simulink model "Attitude_Estimator"  (Simulink 9.0)
settings: Solver=FixedStepDiscrete  StartTime=0.0  StopTime=tsim  FixedStep=te  RelTol=1e-3
values from neighbouring files (symbols this model uses):
  FILTER_KI = 0.1    [Attitude_Estimator_parameters.m]
  FILTER_KP = 1    [Attitude_Estimator_parameters.m]
  Gravity_Err_Threshold = 0.01    [Attitude_Estimator_parameters.m]
  Immobility_Threshold = 0.2    [Attitude_Estimator_parameters.m]
  Immobility_Time_Confirmation = 0.5    [Attitude_Estimator_parameters.m]
  Q_EST_INIT = [0 0 0 1]    [Attitude_Estimator_parameters.m]
  te = 0.01    [Attitude_Estimator_parameters.m]
undefined symbols (not defined in the file or in its folder): DiscIntNeverNeededParam
libraries: simulink x5
settings Model: Creator=sam  LastModifiedBy=William  ExtModeTrigDuration=2
settings DataIOCC: SaveFormat=Dataset
settings OptimizationCC: DefaultParameterBehavior=Inlined  DefaultUnderspecifiedDataType=single  PassReuseOutputArgsThreshold=0  LifeSpan=auto  MaxStackSize=64
settings DebuggingCC: UnderspecifiedInitializationDetection=Simplified  MergeDetectMultiDrivingBlocksExec=error  ParameterPrecisionLossMsg=none  ParameterTunabilityLossMsg=error
settings HardwareCC: ProdBitPerPointer=64  ProdBitPerSizeT=64  ProdBitPerPtrDiffT=64  ProdLargestAtomicFloat=Float  ProdIntDivRoundTo=Zero  ProdEndianess=LittleEndian  ProdWordSize=64  ProdHWDeviceType=Intel->x86-64 (Windows64)
settings ModelReferenceCC: PropagateSignalLabelsOutOfModel=on
settings SFSimCC: MATLABDynamicMemAlloc=off
settings RTWCC: GenerateReport=on  Toolchain=Arduino ARM  BuildConfiguration=Faster Runs  LaunchReport=on  RTWCompilerOptimization=on
settings CodeAppCC: ForceParamTrailComments=on  MaxIdLength=95  OperatorAnnotations=on  MATLABSourceComments=on
settings ConfigComp: CovScope=ReferencedModels  CovIncludeTopModel=off  CovSaveName=covdata_decision  CovMetricSettings=dcmw  CovHTMLOptions=-sRT=1 -sVT=0 -aTS=1 -bRG=1 -bTC=1 -hTR=0 -nFC=0 -nFD=1 -scm=1 -bcm=1 -xEv=0 -xEM=0  CovNameIncrementing=on  CovOutputDir=../reports/slcov_output/$ModelName$

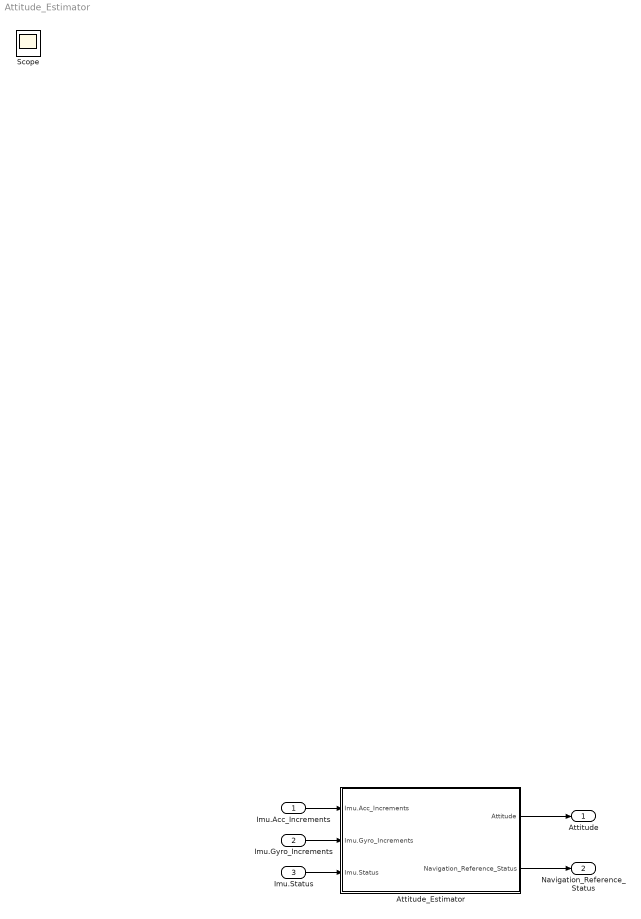
== system Attitude_Estimator ==
  Imu.Acc_Increments : Inport  OutDataTypeStr=single  PortDimensions=3
  Imu.Gyro_Increments : Inport  Port=2  PortDimensions=3
  Imu.Status : Inport  Port=3  PortDimensions=1
  Attitude_Estimator : Subsystem
  Attitude : Outport  PortDimensions=5
  Navigation_Reference_Status : Outport  Port=2  PortDimensions=1
  Scope : Scope
  wires:
  Attitude_Estimator/1(Attitude) -> Attitude/1
  Imu.Acc_Increments/1 -> Attitude_Estimator/1(Imu.Acc_Increments)
  Attitude_Estimator/2(Navigation_Reference_Status) -> Navigation_Reference_Status/1
  Imu.Gyro_Increments/1 -> Attitude_Estimator/2(Imu.Gyro_Increments)
  Imu.Status/1 -> Attitude_Estimator/3(Imu.Status)

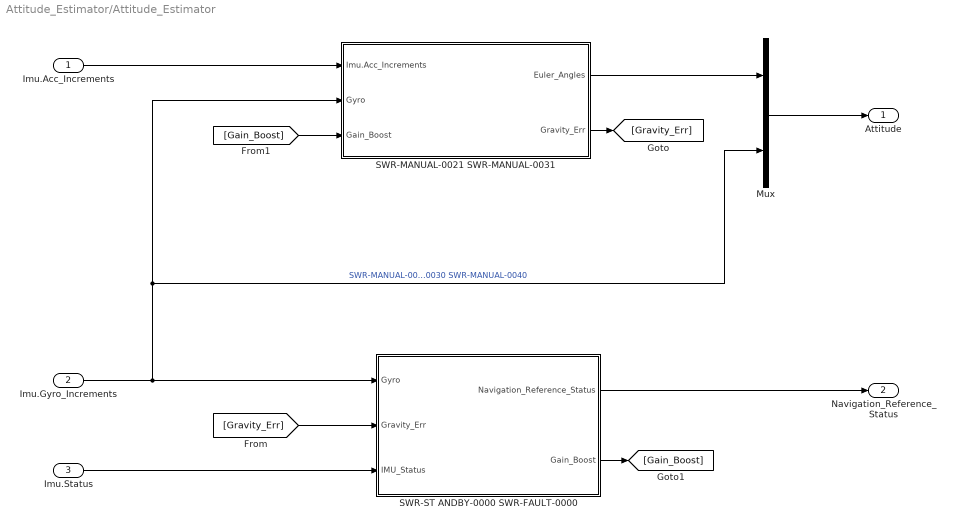
== system Attitude_Estimator/Attitude_Estimator ==
  Imu.Acc_Increments : Inport  OutDataTypeStr=single  PortDimensions=3
  Imu.Gyro_Increments : Inport  Port=2  OutDataTypeStr=single  PortDimensions=3
  Imu.Status : Inport  Port=3  OutDataTypeStr=uint8  PortDimensions=1
  Mux : Mux  Inputs=2
  SWR-MANUAL-0021 SWR-MANUAL-0031 : Subsystem
  SWR-ST	ANDBY-0000 SWR-FAULT-0000 : Subsystem
  Attitude : Outport  OutDataTypeStr=single  PortDimensions=5
  Navigation_Reference_Status : Outport  Port=2  OutDataTypeStr=uint8  PortDimensions=1
  wires:
  Imu.Gyro_Increments/1 -> SWR-ST	ANDBY-0000 SWR-FAULT-0000/1(Gyro), SWR-MANUAL-0021 SWR-MANUAL-0031/2(Gyro), Mux/2  "SWR-MANUAL-0020 SWR-MANUAL-0030 SWR-MANUAL-0040"
  [Gravity_Err] -> SWR-ST	ANDBY-0000 SWR-FAULT-0000/2(Gravity_Err)
  Imu.Status/1 -> SWR-ST	ANDBY-0000 SWR-FAULT-0000/3(IMU_Status)
  SWR-ST	ANDBY-0000 SWR-FAULT-0000/1(Navigation_Reference_Status) -> Navigation_Reference_Status/1
  SWR-ST	ANDBY-0000 SWR-FAULT-0000/2(Gain_Boost) -> [Gain_Boost]
  Mux/1 -> Attitude/1
  Imu.Acc_Increments/1 -> SWR-MANUAL-0021 SWR-MANUAL-0031/1(Imu.Acc_Increments)
  SWR-MANUAL-0021 SWR-MANUAL-0031/2(Gravity_Err) -> [Gravity_Err]
  SWR-MANUAL-0021 SWR-MANUAL-0031/1(Euler_Angles) -> Mux/1
  [Gain_Boost] -> SWR-MANUAL-0021 SWR-MANUAL-0031/3(Gain_Boost)

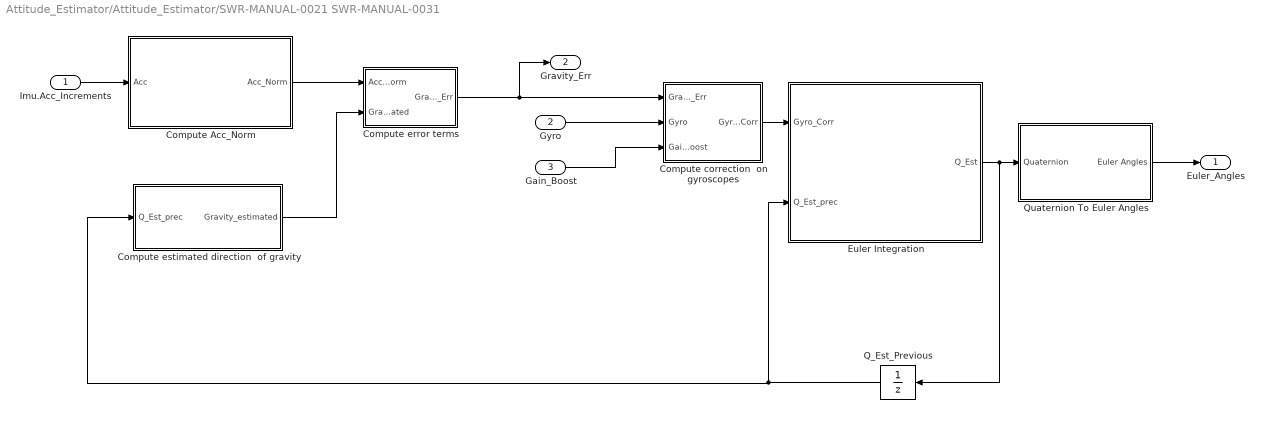
== system Attitude_Estimator/Attitude_Estimator/SWR-MANUAL-0021 SWR-MANUAL-0031 ==
  Imu.Acc_Increments : Inport  OutDataTypeStr=single  PortDimensions=3
  Gyro : Inport  Port=2
  Gain_Boost : Inport  Port=3
  Compute Acc_Norm : Subsystem
  Compute correction  on gyroscopes : Subsystem
  Compute error terms : Subsystem
  Compute estimated direction  of gravity : Subsystem
  Euler Integration : Subsystem
  Q_Est_Previous : UnitDelay  InitialCondition=Q_EST_INIT  SampleTime=te
  Quaternion To Euler Angles : Subsystem
  Euler_Angles : Outport
  Gravity_Err : Outport  Port=2  OutDataTypeStr=single  PortDimensions=3
  wires:
  Euler Integration/1(Q_Est) -> Quaternion To Euler Angles/1(Quaternion), Q_Est_Previous/1
  Compute estimated direction  of gravity/1(Gravity_estimated) -> Compute error terms/2(Gravity_estimated)
  Compute correction  on gyroscopes/1(Gyro_Corr) -> Euler Integration/1(Gyro_Corr)
  Compute Acc_Norm/1(Acc_Norm) -> Compute error terms/1(Acc_Norm)
  Compute error terms/1(Gravity_Err) -> Gravity_Err/1, Compute correction  on gyroscopes/1(Gravity_Err)
  Imu.Acc_Increments/1 -> Compute Acc_Norm/1(Acc)
  Q_Est_Previous/1 -> Compute estimated direction  of gravity/1(Q_Est_prec), Euler Integration/2(Q_Est_prec)
  Quaternion To Euler Angles/1(Euler Angles) -> Euler_Angles/1
  Gain_Boost/1 -> Compute correction  on gyroscopes/3(Gain_Boost)
  Gyro/1 -> Compute correction  on gyroscopes/2(Gyro)

== system Attitude_Estimator/Attitude_Estimator/SWR-ST	ANDBY-0000 SWR-FAULT-0000 ==
  Gyro : Inport
  Gravity_Err : Inport  Port=2
  IMU_Status : Inport  Port=3
  SWR-ST	ANDBY-0000 SWR-FAULT-0000 : Subsystem
  SWR-STANDBY-0000 : Subsystem
  Navigation_Reference_Status : Outport
  Gain_Boost : Outport  Port=2  PortDimensions=1
  wires:
  Gyro/1 -> SWR-STANDBY-0000/2(Gyro)
  Gravity_Err/1 -> SWR-STANDBY-0000/3(Gravity_Err)
  SWR-STANDBY-0000/2(Gain_Boost) -> Gain_Boost/1
  IMU_Status/1 -> SWR-STANDBY-0000/1(IMU_Status), SWR-ST	ANDBY-0000 SWR-FAULT-0000/1(Imu_Status)
  SWR-STANDBY-0000/1(Alignment_OK) -> SWR-ST	ANDBY-0000 SWR-FAULT-0000/2(Alignment_OK)
  SWR-ST	ANDBY-0000 SWR-FAULT-0000/1(Navigation_Reference_Status) -> Navigation_Reference_Status/1

== system Attitude_Estimator/Attitude_Estimator/SWR-MANUAL-0021 SWR-MANUAL-0031/Compute Acc_Norm ==
  Acc : Inport  PortDimensions=3
  Normalize 3D Vector : Subsystem
  Acc_Norm : Outport  OutDataTypeStr=single  PortDimensions=3
  wires:
  Acc/1 -> Normalize 3D Vector/1(Acc)
  Normalize 3D Vector/1(Acc_Norm) -> Acc_Norm/1

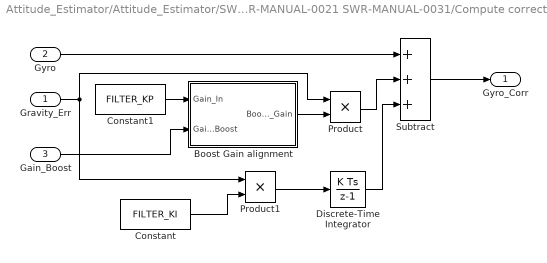
== system Attitude_Estimator/Attitude_Estimator/SWR-MANUAL-0021 SWR-MANUAL-0031/Compute correction  on gyroscopes ==
  Gravity_Err : Inport  PortDimensions=3
  Gyro : Inport  Port=2  PortDimensions=3
  Gain_Boost : Inport  Port=3  PortDimensions=1
  Boost Gain alignment : Subsystem
  Constant : Constant  Value=FILTER_KI  OutDataTypeStr=single
  Constant1 : Constant  Value=FILTER_KP  OutDataTypeStr=single
  Discrete-Time Integrator : DiscreteIntegrator  InitialConditionSetting=State (most efficient)  SampleTime=te  ICPrevOutput=DiscIntNeverNeededParam  ICPrevScaledInput=DiscIntNeverNeededParam
  Product : Product
  Product1 : Product
  Subtract : Sum  Inputs=+++
  Gyro_Corr : Outport  PortDimensions=3
  wires:
  Gyro/1 -> Subtract/1
  Subtract/1 -> Gyro_Corr/1
  Gravity_Err/1 -> Product1/1, Product/1
  Product/1 -> Subtract/2
  Constant/1 -> Product1/2
  Product1/1 -> Discrete-Time Integrator/1
  Discrete-Time Integrator/1 -> Subtract/3
  Boost Gain alignment/1(Boosted_Gain) -> Product/2
  Constant1/1 -> Boost Gain alignment/1(Gain_In)
  Gain_Boost/1 -> Boost Gain alignment/2(Gain_Boost)

== system Attitude_Estimator/Attitude_Estimator/SWR-MANUAL-0021 SWR-MANUAL-0031/Compute error terms ==
  Acc_Norm : Inport  PortDimensions=3
  Gravity_estimated : Inport  Port=2  PortDimensions=3
  Cross Product : Subsystem
  Gravity_Err : Outport  PortDimensions=3
  wires:
  Gravity_estimated/1 -> Cross Product/1(Vec1)
  Acc_Norm/1 -> Cross Product/2(Vec2)
  Cross Product/1(Prod_Vec) -> Gravity_Err/1

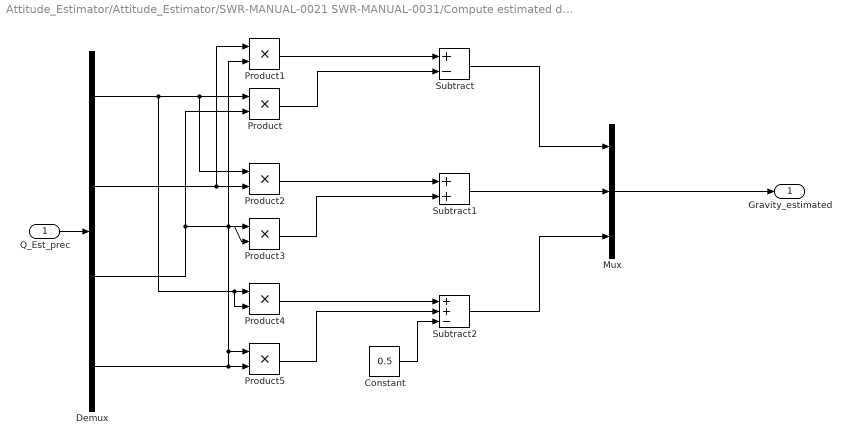
== system Attitude_Estimator/Attitude_Estimator/SWR-MANUAL-0021 SWR-MANUAL-0031/Compute estimated direction  of gravity ==
  Q_Est_prec : Inport  PortDimensions=4
  Constant : Constant  Value=0.5  OutDataTypeStr=single
  Demux : Demux
  Mux : Mux  Inputs=3
  Product{,1..5} (6 alike) : Product
  Subtract : Sum  Inputs=+-
  Subtract1 : Sum
  Subtract2 : Sum  Inputs=++-
  Gravity_estimated : Outport
  wires:
  Q_Est_prec/1 -> Demux/1
  Demux/2 -> Product2/2, Product1/1
  Demux/4 -> Product5/1, Product3/2, Product1/2, Product5/2
  Demux/1 -> Product/1, Product2/1, Product4/2, Product4/1
  Demux/3 -> Product/2, Product3/1
  Product1/1 -> Subtract/1
  Product/1 -> Subtract/2
  Product2/1 -> Subtract1/1
  Product3/1 -> Subtract1/2
  Product4/1 -> Subtract2/1
  Product5/1 -> Subtract2/2
  Constant/1 -> Subtract2/3
  Subtract/1 -> Mux/1
  Subtract1/1 -> Mux/2
  Subtract2/1 -> Mux/3
  Mux/1 -> Gravity_estimated/1

== system Attitude_Estimator/Attitude_Estimator/SWR-MANUAL-0021 SWR-MANUAL-0031/Euler Integration ==
  Gyro_Corr : Inport  PortDimensions=3
  Q_Est_prec : Inport  Port=2  PortDimensions=4
  Add : Sum
  Compute Kinematic Propagation Quaternion : Subsystem
  Compute Unit Quaternion : Subsystem
  Gain : Gain  Gain=0.5*te  OutDataTypeStr=single
  Q_Est : Outport  PortDimensions=4
  wires:
  Compute Unit Quaternion/1(Qn) -> Q_Est/1
  Q_Est_prec/1 -> Add/1, Compute Kinematic Propagation Quaternion/1(Q_Est_Prec)
  Gyro_Corr/1 -> Compute Kinematic Propagation Quaternion/2(W_F inal)
  Compute Kinematic Propagation Quaternion/1(Kin_Prop_Quat) -> Gain/1
  Gain/1 -> Add/2
  Add/1 -> Compute Unit Quaternion/1(Q)

== system Attitude_Estimator/Attitude_Estimator/SWR-MANUAL-0021 SWR-MANUAL-0031/Quaternion To Euler Angles ==
  Quaternion : Inport  PortDimensions=4
  Compute Pitch : Subsystem
  "Compute Roll " : Subsystem
  Mux : Mux  Inputs=2
  Euler Angles : Outport  PortDimensions=2
  wires:
  Mux/1 -> Euler Angles/1
  "Compute Roll "/1(Roll) -> Mux/1
  Quaternion/1 -> Compute Pitch/1(Quaternion), "Compute Roll "/1(Quaternion)
  Compute Pitch/1(Pitch) -> Mux/2

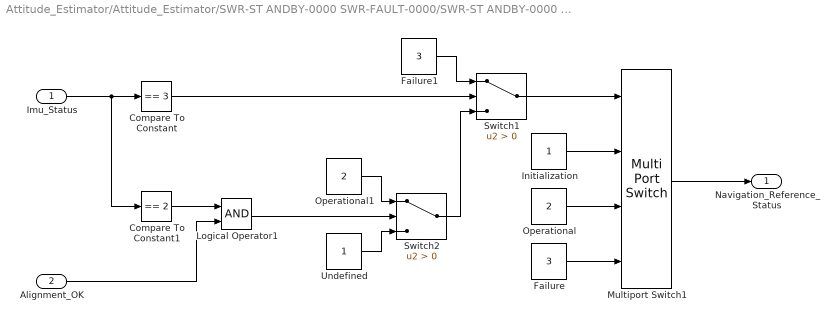
== system Attitude_Estimator/Attitude_Estimator/SWR-ST	ANDBY-0000 SWR-FAULT-0000/SWR-ST	ANDBY-0000 SWR-FAULT-0000 ==
  Imu_Status : Inport
  Alignment_OK : Inport  Port=2
  Compare To Constant : simulink/Logic and Bit Operations/Compare To Constant  relop===  const=3  OutDataTypeStr=boolean
  Compare To Constant1 : simulink/Logic and Bit Operations/Compare To Constant  relop===  const=2  OutDataTypeStr=boolean
  Failure : Constant  Value=3  OutDataTypeStr=uint8
  Failure1 : Constant  Value=3  OutDataTypeStr=uint8
  Initialization : Constant  OutDataTypeStr=uint8
  Logical Operator1 : Logic  AllPortsSameDT=off  OutDataTypeStr=boolean
  Multiport Switch1 : MultiPortSwitch  DiagnosticForDefault=None
  Operational : Constant  Value=2  OutDataTypeStr=uint8
  Operational1 : Constant  Value=2  OutDataTypeStr=uint8
  Switch1 : Switch  Criteria=u2 > Threshold
  Switch2 : Switch  Criteria=u2 > Threshold
  Undefined : Constant  OutDataTypeStr=uint8
  Navigation_Reference_Status : Outport
  wires:
  Logical Operator1/1 -> Switch2/2
  Compare To Constant1/1 -> Logical Operator1/1
  Undefined/1 -> Switch2/3
  Switch1/1 -> Multiport Switch1/1
  Failure1/1 -> Switch1/1
  Operational1/1 -> Switch2/1
  Switch2/1 -> Switch1/3
  Multiport Switch1/1 -> Navigation_Reference_Status/1
  Initialization/1 -> Multiport Switch1/2
  Operational/1 -> Multiport Switch1/3
  Failure/1 -> Multiport Switch1/4
  Alignment_OK/1 -> Logical Operator1/2
  Compare To Constant/1 -> Switch1/2
  Imu_Status/1 -> Compare To Constant/1, Compare To Constant1/1

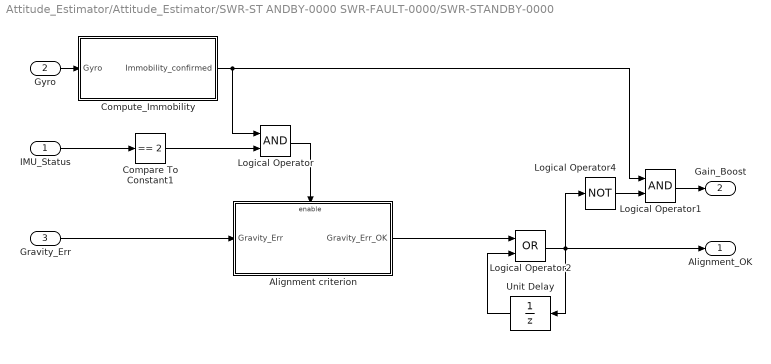
== system Attitude_Estimator/Attitude_Estimator/SWR-ST	ANDBY-0000 SWR-FAULT-0000/SWR-STANDBY-0000 ==
  IMU_Status : Inport
  Gyro : Inport  Port=2
  Gravity_Err : Inport  Port=3
  Alignment criterion : Subsystem  TreatAsAtomicUnit=on
  Compare To Constant1 : simulink/Logic and Bit Operations/Compare To Constant  relop===  const=2  OutDataTypeStr=boolean
  Compute_Immobility : Subsystem
  Logical Operator : Logic  AllPortsSameDT=off  OutDataTypeStr=boolean
  Logical Operator1 : Logic  AllPortsSameDT=off  OutDataTypeStr=boolean
  Logical Operator2 : Logic  Operator=OR  AllPortsSameDT=off  OutDataTypeStr=boolean
  Logical Operator4 : Logic  Operator=NOT  AllPortsSameDT=off  OutDataTypeStr=boolean
  Unit Delay : UnitDelay  SampleTime=te
  Alignment_OK : Outport  PortDimensions=1
  Gain_Boost : Outport  Port=2  PortDimensions=1
  wires:
  Gyro/1 -> Compute_Immobility/1(Gyro)
  Compute_Immobility/1(Immobility_confirmed) -> Logical Operator1/1, Logical Operator/1
  Logical Operator2/1 -> Alignment_OK/1, Unit Delay/1, Logical Operator4/1
  Unit Delay/1 -> Logical Operator2/2
  Gravity_Err/1 -> Alignment criterion/1(Gravity_Err)
  Logical Operator1/1 -> Gain_Boost/1
  Logical Operator4/1 -> Logical Operator1/2
  Logical Operator/1 -> Alignment criterion/Enable
  IMU_Status/1 -> Compare To Constant1/1
  Compare To Constant1/1 -> Logical Operator/2
  Alignment criterion/1(Gravity_Err_OK) -> Logical Operator2/1

== system Attitude_Estimator/Attitude_Estimator/SWR-MANUAL-0021 SWR-MANUAL-0031/Compute Acc_Norm/Normalize 3D Vector ==
  Acc : Inport  PortDimensions=3
  Compare To Constant : simulink/Logic and Bit Operations/Compare To Constant  relop===  const=0.0  OutDataTypeStr=boolean
  Constant : Constant  OutDataTypeStr=single
  Divide : Product  Inputs=*/
  Switch : Switch  Criteria=u2 > Threshold
  Vect 3D Norm : Subsystem
  Acc_Norm : Outport  PortDimensions=3
  wires:
  Acc/1 -> Vect 3D Norm/1(Vect_3D), Divide/1
  Vect 3D Norm/1(Vect_3D_Norm) -> Compare To Constant/1, Switch/3
  Compare To Constant/1 -> Switch/2
  Switch/1 -> Divide/2
  Divide/1 -> Acc_Norm/1
  Constant/1 -> Switch/1

== system Attitude_Estimator/Attitude_Estimator/SWR-MANUAL-0021 SWR-MANUAL-0031/Compute correction  on gyroscopes/Boost Gain alignment ==
  Gain_In : Inport  PortDimensions=1
  Gain_Boost : Inport  Port=2  PortDimensions=1
  Gain : Gain  Gain=10
  Switch : Switch  Criteria=u2 > Threshold
  Boosted_Gain : Outport  PortDimensions=1
  wires:
  Switch/1 -> Boosted_Gain/1
  Gain_In/1 -> Gain/1, Switch/3
  Gain_Boost/1 -> Switch/2
  Gain/1 -> Switch/1

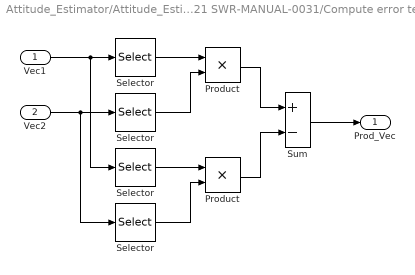
== system Attitude_Estimator/Attitude_Estimator/SWR-MANUAL-0021 SWR-MANUAL-0031/Compute error terms/Cross Product ==
  Vec1 : Inport  PortDimensions=3
  Vec2 : Inport  Port=2  PortDimensions=3
  " Selector " : Selector  IndexMode=Zero-based  InputPortWidth=3  IndexOptions=Index vector (dialog)  Indices=[1 2 0]  OutputSizes=1
  Product : Product  RndMeth=Zero  InputSameDT=on  OutDataTypeStr=Inherit: Same as first input
  "Product " : Product  RndMeth=Zero  InputSameDT=on  OutDataTypeStr=Inherit: Same as first input
  Selector : Selector  IndexMode=Zero-based  InputPortWidth=3  IndexOptions=Index vector (dialog)  Indices=[1 2 0]  OutputSizes=1
  "Selector " : Selector  IndexMode=Zero-based  InputPortWidth=3  IndexOptions=Index vector (dialog)  Indices=[2 0 1]  OutputSizes=1
  "Selector  " : Selector  IndexMode=Zero-based  InputPortWidth=3  IndexOptions=Index vector (dialog)  Indices=[2 0 1]  OutputSizes=1
  Sum : Sum  Inputs=+-  InputSameDT=on  OutDataTypeStr=Inherit: Same as first input
  Prod_Vec : Outport  PortDimensions=3
  wires:
  "Selector  "/1 -> "Product "/1
  Selector/1 -> Product/1
  Sum/1 -> Prod_Vec/1
  " Selector "/1 -> "Product "/2
  "Product "/1 -> Sum/2
  "Selector "/1 -> Product/2
  Product/1 -> Sum/1
  Vec1/1 -> "Selector  "/1, Selector/1
  Vec2/1 -> " Selector "/1, "Selector "/1

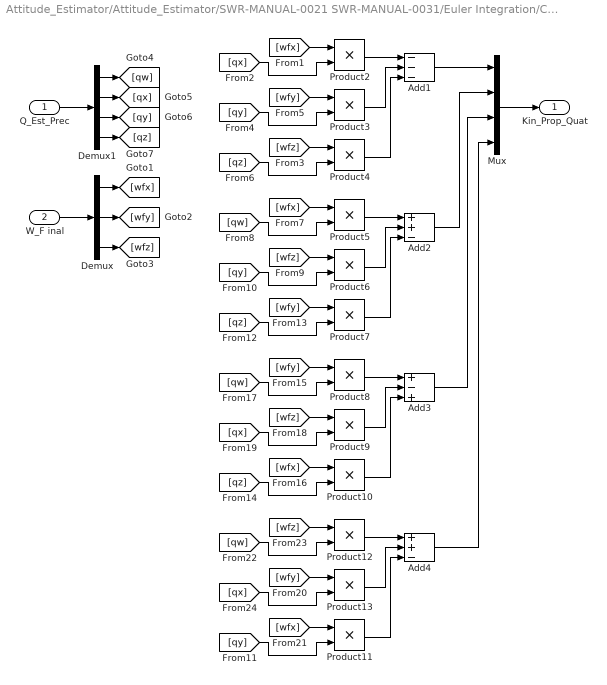
== system Attitude_Estimator/Attitude_Estimator/SWR-MANUAL-0021 SWR-MANUAL-0031/Euler Integration/Compute Kinematic Propagation Quaternion ==
  Q_Est_Prec : Inport  PortDimensions=4
  W_F inal : Inport  Port=2  PortDimensions=3
  Add1 : Sum  Inputs=---
  Add2 : Sum  Inputs=++-
  Add3 : Sum  Inputs=+-+
  Add4 : Sum  Inputs=++-
  Demux : Demux  Outputs=3
  Demux1 : Demux
  Mux : Mux
  Product{2..13} (12 alike) : Product
  Kin_Prop_Quat : Outport  PortDimensions=4
  wires:
  [wfx] -> Product11/1
  [wfz] -> Product12/1
  Demux1/3 -> [qy]
  Add2/1 -> Mux/2
  [wfx] -> Product10/1
  Product10/1 -> Add3/3
  [wfz] -> Product6/1
  Demux1/2 -> [qx]
  [wfy] -> Product7/1
  Demux/3 -> [wfz]
  Product11/1 -> Add4/3
  [qw] -> Product8/2
  Demux/1 -> [wfx]
  Add4/1 -> Mux/4
  Product5/1 -> Add2/1
  Q_Est_Prec/1 -> Demux1/1
  [wfx] -> Product2/1
  Add3/1 -> Mux/3
  Product7/1 -> Add2/3
  [wfz] -> Product9/1
  Product4/1 -> Add1/3
  [qz] -> Product7/2
  Product9/1 -> Add3/2
  Product3/1 -> Add1/2
  Product2/1 -> Add1/1
  Product6/1 -> Add2/2
  [qw] -> Product12/2
  Demux1/1 -> [qw]
  [qy] -> Product11/2
  [qy] -> Product6/2
  Product12/1 -> Add4/1
  [qx] -> Product9/2
  [qz] -> Product10/2
  Demux1/4 -> [qz]
  [wfy] -> Product13/1
  Product8/1 -> Add3/1
  [qw] -> Product5/2
  [qy] -> Product3/2
  [wfx] -> Product5/1
  Product13/1 -> Add4/2
  Add1/1 -> Mux/1
  Mux/1 -> Kin_Prop_Quat/1
  [qx] -> Product13/2
  Demux/2 -> [wfy]
  W_F inal/1 -> Demux/1
  [qx] -> Product2/2
  [wfy] -> Product8/1
  [wfy] -> Product3/1
  [wfz] -> Product4/1
  [qz] -> Product4/2

== system Attitude_Estimator/Attitude_Estimator/SWR-MANUAL-0021 SWR-MANUAL-0031/Euler Integration/Compute Unit Quaternion ==
  Q : Inport  PortDimensions=4
  Compare To Constant : simulink/Logic and Bit Operations/Compare To Constant  relop===  const=0  OutDataTypeStr=uint8
  Constant : Constant  OutDataTypeStr=single
  Divide : Product  Inputs=*/  OutDataTypeStr=Inherit: Same as first input
  Quaternion Norm : Subsystem
  Switch : Switch  Criteria=u2 > Threshold
  Qn : Outport  PortDimensions=4
  wires:
  Q/1 -> Divide/1, Quaternion Norm/1(Q)
  Divide/1 -> Qn/1
  Switch/1 -> Divide/2
  Compare To Constant/1 -> Switch/2
  Quaternion Norm/1(Q_Norm) -> Compare To Constant/1, Switch/3
  Constant/1 -> Switch/1

== system Attitude_Estimator/Attitude_Estimator/SWR-MANUAL-0021 SWR-MANUAL-0031/Quaternion To Euler Angles/Compute Pitch ==
  Quaternion : Inport
  2*(qw*qy-qz*qx) : Subsystem
  Asin : Trigonometry  Operator=asin
  Pitch : Outport
  wires:
  2*(qw*qy-qz*qx)/1(First term) -> Asin/1
  Quaternion/1 -> 2*(qw*qy-qz*qx)/1(Quaternion)
  Asin/1 -> Pitch/1

== system Attitude_Estimator/Attitude_Estimator/SWR-MANUAL-0021 SWR-MANUAL-0031/Quaternion To Euler Angles/Compute Roll  ==
  Quaternion : Inport
  1 - 2*(qx² + qy²) : Subsystem
  2*(qw*qx + qy*qz) : Subsystem
  Atan2 : Trigonometry  Operator=atan2
  Roll : Outport
  wires:
  Atan2/1 -> Roll/1
  Quaternion/1 -> 1 - 2*(qx² + qy²)/1(Quaternion), 2*(qw*qx + qy*qz)/1(Quaternion)
  1 - 2*(qx² + qy²)/1(Second term) -> Atan2/2
  2*(qw*qx + qy*qz)/1(First term) -> Atan2/1

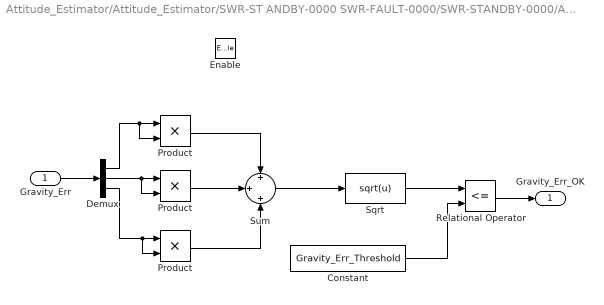
== system Attitude_Estimator/Attitude_Estimator/SWR-ST	ANDBY-0000 SWR-FAULT-0000/SWR-STANDBY-0000/Alignment criterion ==
  Gravity_Err : Inport  PortDimensions=3
  Enable : EnablePort
  Constant : Constant  Value=Gravity_Err_Threshold  OutDataTypeStr=single
  Demux : Demux  Outputs=3
  Product : Product
  "Product " : Product
  "Product  " : Product
  Relational Operator : RelationalOperator  Operator=<=  OutDataTypeStr=boolean  RndMeth=Simplest
  Sqrt : Fcn  Expr=sqrt(u)
  Sum : Sum  Inputs=+|+|+
  Gravity_Err_OK : Outport  OutputWhenDisabled=reset  InitialOutput=false
  wires:
  Product/1 -> Sum/1
  Sum/1 -> Sqrt/1
  "Product "/1 -> Sum/2
  Demux/3 -> "Product  "/2, "Product  "/1
  "Product  "/1 -> Sum/3
  Demux/1 -> Product/1, Product/2
  Gravity_Err/1 -> Demux/1
  Demux/2 -> "Product "/2, "Product "/1
  Sqrt/1 -> Relational Operator/1
  Constant/1 -> Relational Operator/2
  Relational Operator/1 -> Gravity_Err_OK/1

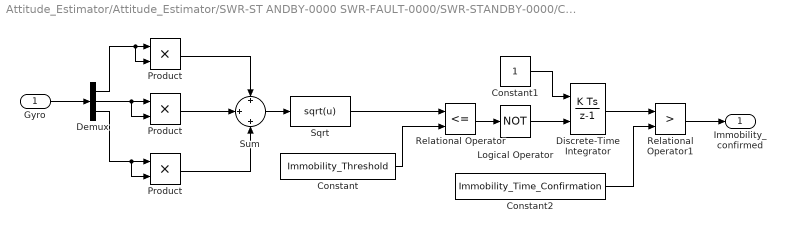
== system Attitude_Estimator/Attitude_Estimator/SWR-ST	ANDBY-0000 SWR-FAULT-0000/SWR-STANDBY-0000/Compute_Immobility ==
  Gyro : Inport  PortDimensions=3
  Constant : Constant  Value=Immobility_Threshold  OutDataTypeStr=single
  Constant1 : Constant  OutDataTypeStr=single
  Constant2 : Constant  Value=Immobility_Time_Confirmation  OutDataTypeStr=single
  Demux : Demux  Outputs=3
  Discrete-Time Integrator : DiscreteIntegrator  ExternalReset=level  InitialConditionSetting=State (most efficient)  SampleTime=te  ICPrevOutput=DiscIntNeverNeededParam  ICPrevScaledInput=DiscIntNeverNeededParam
  Logical Operator : Logic  Operator=NOT  AllPortsSameDT=off  OutDataTypeStr=boolean
  Product : Product
  "Product " : Product
  "Product  " : Product
  Relational Operator : RelationalOperator  Operator=<=  OutDataTypeStr=boolean  RndMeth=Simplest
  Relational Operator1 : RelationalOperator  Operator=>  OutDataTypeStr=boolean  RndMeth=Simplest
  Sqrt : Fcn  Expr=sqrt(u)
  Sum : Sum  Inputs=+|+|+
  Immobility_confirmed : Outport  PortDimensions=1
  wires:
  Sum/1 -> Sqrt/1
  Demux/3 -> "Product  "/2, "Product  "/1
  "Product  "/1 -> Sum/3
  "Product "/1 -> Sum/2
  Demux/2 -> "Product "/2, "Product "/1
  Product/1 -> Sum/1
  Gyro/1 -> Demux/1
  Demux/1 -> Product/2, Product/1
  Sqrt/1 -> Relational Operator/1
  Constant/1 -> Relational Operator/2
  Relational Operator/1 -> Logical Operator/1
  Constant1/1 -> Discrete-Time Integrator/1
  Discrete-Time Integrator/1 -> Relational Operator1/1
  Constant2/1 -> Relational Operator1/2
  Relational Operator1/1 -> Immobility_confirmed/1
  Logical Operator/1 -> Discrete-Time Integrator/2

== system Attitude_Estimator/Attitude_Estimator/SWR-MANUAL-0021 SWR-MANUAL-0031/Compute Acc_Norm/Normalize 3D Vector/Vect 3D Norm ==
  Vect_3D : Inport  PortDimensions=3
  Demux : Demux  Outputs=3
  Product : Product
  "Product " : Product
  "Product  " : Product
  Sqrt : Fcn  Expr=sqrt(u)
  Sum : Sum  Inputs=+|+|+  OutDataTypeStr=Inherit: Inherit via back propagation
  Vect_3D_Norm : Outport  OutDataTypeStr=single  PortDimensions=1
  wires:
  Sqrt/1 -> Vect_3D_Norm/1
  Sum/1 -> Sqrt/1
  Demux/3 -> "Product  "/2, "Product  "/1
  "Product  "/1 -> Sum/3
  "Product "/1 -> Sum/2
  Demux/2 -> "Product "/2, "Product "/1
  Product/1 -> Sum/1
  Vect_3D/1 -> Demux/1
  Demux/1 -> Product/2, Product/1

== system Attitude_Estimator/Attitude_Estimator/SWR-MANUAL-0021 SWR-MANUAL-0031/Euler Integration/Compute Unit Quaternion/Quaternion Norm ==
  Q : Inport  PortDimensions=4
  " Product " : Product
  " Product  " : Product
  Demux : Demux
  Product : Product
  "Product " : Product
  Sqrt1 : Fcn  Expr=sqrt(u)
  Sum : Sum  Inputs=++++  OutDataTypeStr=Inherit: Inherit via back propagation
  Q_Norm : Outport  OutDataTypeStr=single  PortDimensions=1
  wires:
  Q/1 -> Demux/1
  Demux/1 -> Product/2, Product/1
  Demux/2 -> "Product "/2, "Product "/1
  Demux/3 -> " Product "/2, " Product "/1
  Demux/4 -> " Product  "/2, " Product  "/1
  Product/1 -> Sum/1
  "Product "/1 -> Sum/2
  " Product "/1 -> Sum/3
  " Product  "/1 -> Sum/4
  Sum/1 -> Sqrt1/1
  Sqrt1/1 -> Q_Norm/1

== system Attitude_Estimator/Attitude_Estimator/SWR-MANUAL-0021 SWR-MANUAL-0031/Quaternion To Euler Angles/Compute Pitch/2*(qw*qy-qz*qx) ==
  Quaternion : Inport
  Add : Sum  Inputs=+-  OutDataTypeStr=Inherit: Same as first input
  Demux : Demux
  Gain1 : Gain  Gain=2  OutDataTypeStr=single  ParamDataTypeStr=Inherit: Same as input
  qw*qy : Product  OutDataTypeStr=Inherit: Same as first input
  qx*qz : Product  OutDataTypeStr=Inherit: Same as first input
  First term : Outport
  wires:
  qx*qz/1 -> Add/2
  Gain1/1 -> First term/1
  Quaternion/1 -> Demux/1
  Add/1 -> Gain1/1
  Demux/1 -> qw*qy/1
  qw*qy/1 -> Add/1
  Demux/4 -> qx*qz/2
  Demux/3 -> qw*qy/2
  Demux/2 -> qx*qz/1

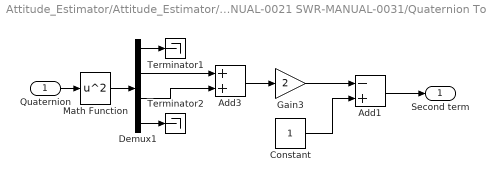
== system Attitude_Estimator/Attitude_Estimator/SWR-MANUAL-0021 SWR-MANUAL-0031/Quaternion To Euler Angles/Compute Roll /1 - 2*(qx² + qy²) ==
  Quaternion : Inport
  Add1 : Sum  Inputs=-+
  Add3 : Sum
  Constant : Constant  OutDataTypeStr=single
  Demux1 : Demux
  Gain3 : Gain  Gain=2
  Math Function : Math  Operator=square
  Terminator1 : Terminator
  Terminator2 : Terminator
  Second term : Outport
  wires:
  Add1/1 -> Second term/1
  Math Function/1 -> Demux1/1
  Add3/1 -> Gain3/1
  Gain3/1 -> Add1/1
  Demux1/4 -> Terminator2/1
  Demux1/3 -> Add3/2
  Constant/1 -> Add1/2
  Quaternion/1 -> Math Function/1
  Demux1/2 -> Add3/1
  Demux1/1 -> Terminator1/1

== system Attitude_Estimator/Attitude_Estimator/SWR-MANUAL-0021 SWR-MANUAL-0031/Quaternion To Euler Angles/Compute Roll /2*(qw*qx + qy*qz) ==
  Quaternion : Inport
  Add : Sum
  Demux : Demux
  Gain1 : Gain  Gain=2  OutDataTypeStr=single
  qw*qx : Product
  qy*qz : Product
  First term : Outport
  wires:
  Demux/4 -> qy*qz/2
  qw*qx/1 -> Add/1
  Demux/1 -> qw*qx/1
  Demux/3 -> qy*qz/1
  Add/1 -> Gain1/1
  Demux/2 -> qw*qx/2
  Quaternion/1 -> Demux/1
  Gain1/1 -> First term/1
  qy*qz/1 -> Add/2
